simulink model "controle_discreto"  (R2022a)
settings: Solver=FixedStepDiscrete  StartTime=0.0  StopTime=30  FixedStep=delta_time  RelTol=1e-3
undefined symbols (not defined in the file or in its folder): Cden, Cnum, Hden, Hnum, sym2poly
settings Model: Creator=phcs  LastModifiedBy=phcs

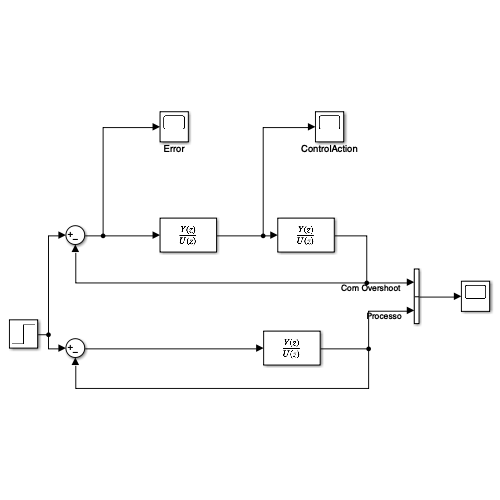
[thumbnail: Simulink's stored preview of the top-level diagram]
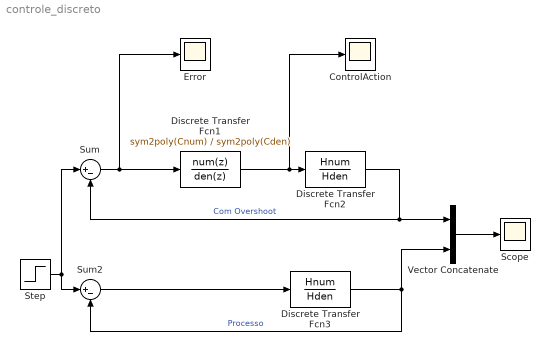
== system controle_discreto ==
  ControlAction : Scope
  Discrete Transfer Fcn1 : DiscreteTransferFcn  Numerator=sym2poly(Cnum)  Denominator=sym2poly(Cden)
  Discrete Transfer Fcn2 : DiscreteTransferFcn  Numerator=Hnum  Denominator=Hden
  Discrete Transfer Fcn3 : DiscreteTransferFcn  Numerator=Hnum  Denominator=Hden
  Error : Scope
  Scope : Scope
  Step : Step  SampleTime=0
  Sum : Sum  Inputs=|+-
  Sum2 : Sum  Inputs=|+-
  Vector Concatenate : Concatenate
  wires:
  Discrete Transfer Fcn2/1 -> Vector Concatenate/1, Sum/2  "Com Overshoot"
  Vector Concatenate/1 -> Scope/1
  Sum2/1 -> Discrete Transfer Fcn3/1
  Discrete Transfer Fcn3/1 -> Vector Concatenate/2, Sum2/2  "Processo"
  Step/1 -> Sum2/1, Sum/1
  Discrete Transfer Fcn1/1 -> Discrete Transfer Fcn2/1, ControlAction/1
  Sum/1 -> Error/1, Discrete Transfer Fcn1/1
